simulink model "direct_event1_eg_2"  (R2018a)
settings: Solver=VariableStepAuto  StartTime=0.0  StopTime=10.0  RelTol=1e-3
settings Model: Creator=86188  LastModifiedBy=BEAR

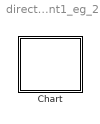
== system direct_event1_eg_2 ==
  Chart : Stateflow chart  TreatAsAtomicUnit=on

== stateflow chart direct_event1_eg_2/Chart ==
  state A [parallel]
    settings: executionOrder=1
    state A2
    state A1
    (default) -> A1
    A1 -> A2 : [data==1]{send(E_one,B)}
    A2 -> A1 : E_two
  state B [parallel]
    settings: executionOrder=2
    state B2
    state B1
    (default) -> B1
    B1 -> B2 : E_one
    B2 -> B1 : E_two
  data: data local double =1
  events: E_one local FUNCTION_CALL_EVENT; E_two local FUNCTION_CALL_EVENT
